simulink model "Inverter0"  (R2021a)
settings: Solver=VariableStepAuto  StartTime=0.0  StopTime=10.0  RelTol=1e-3
settings Model: Creator=Utkarsh Anand  LastModifiedBy=Utkarsh Anand
settings DataIOCC: SaveOutput=off  SaveTime=off

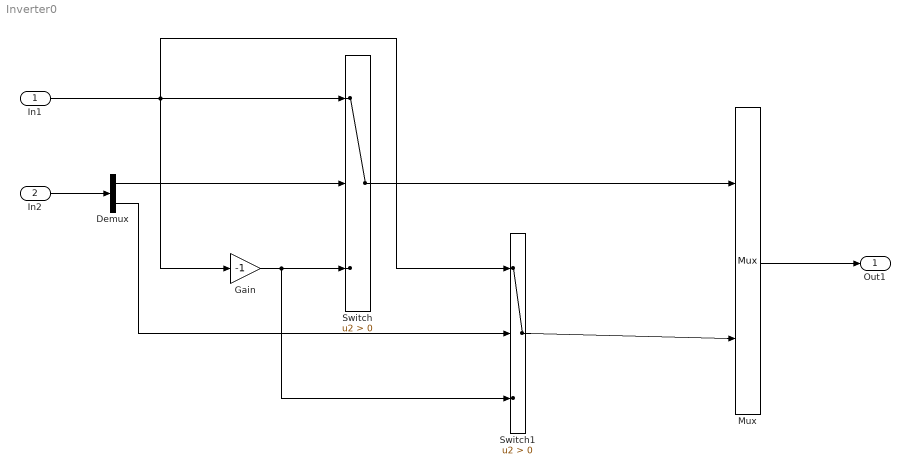
== system Inverter0 ==
  In1 : Inport  OutDataTypeStr=double  PortDimensions=1  SampleTime=0
  In2 : Inport  Port=2  OutDataTypeStr=double  PortDimensions=2  SampleTime=0
  Demux : Demux  Outputs=2
  Gain : Gain  Gain=-1
  Mux : Mux  Inputs=2
  Switch : Switch  Criteria=u2 > Threshold
  Switch1 : Switch  Criteria=u2 > Threshold
  Out1 : Outport  OutDataTypeStr=double  PortDimensions=2  SampleTime=0
  wires:
  Switch1/1 -> Mux/2
  Gain/1 -> Switch1/3, Switch/3
  Demux/2 -> Switch1/2
  In1/1 -> Switch/1, Gain/1, Switch1/1
  Switch/1 -> Mux/1
  Mux/1 -> Out1/1
  Demux/1 -> Switch/2
  In2/1 -> Demux/1
